simulink model "mex_test"  (R2013a)
settings: Solver=FixedStepDiscrete  StartTime=0.0  StopTime=100  FixedStep=1  RelTol=1e-3
undefined symbols (not defined in the file): serial
libraries: instrumentlib x2, aerolibanimutils x1
settings Model: Creator=Admin  LastModifiedBy=Admin
settings HardwareCC: ProdIntDivRoundTo=Zero  ProdEndianess=LittleEndian  ProdHWDeviceType=Generic->32-bit x86 compatible
settings RTWCC: ProcessScript=grt_make_rtw_hook  RTWCompilerOptimization=On
settings CodeAppCC: MaxIdLength=95

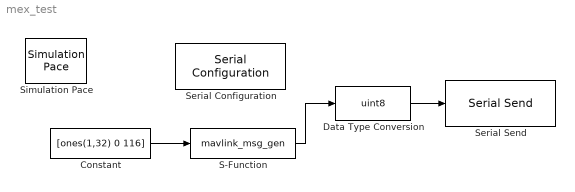
== system mex_test ==
  Constant : Constant  Value=[ones(1,32) 0 116]
  Data Type Conversion : DataTypeConversion  OutDataTypeStr=uint8
  S-Function : S-Function  FunctionName=mavlink_msg_gen  EnableBusSupport=off  mask{mask_msg_id=0}
      mask prompts: mask_msg_id "msg_id"
  Serial Configuration : instrumentlib/Serial Configuration  Priority=-200000  ComPortMenu=COM4  ComPort=COM4  ObjConstructor=serial('COM4');  BaudRate=115200  DataBits=8  Parity=none  StopBits=1  FlowControl=none  Timeout=10  ByteOrder=LittleEndian
  Serial Send : instrumentlib/Serial Send  ComPortMenu=COM4  ComPort=COM4  ObjConstructor=serial('COM4');  Terminator=<none>  EnableBlockingMode=on
  Simulation Pace : aerolibanimutils/Simulation Pace  SimulationPace=1.2  SleepMode=MATLAB Thread  OutputPaceError=off  SampleTime=-1
      settings: AttributesFormatString=%<SimulationPace> sec/sec
  wires:
  Constant/1 -> S-Function/1
  S-Function/1 -> Data Type Conversion/1
  Data Type Conversion/1 -> Serial Send/1
